simulink subsystem "In_Plane_ModelArchitecture"  (R2025b)
settings: Solver=VariableStepAuto  StartTime=0.0  StopTime=10.0  RelTol=1e-3
undefined symbols (not defined in the file or in its folder): AeroLiftCff, AeroLongDrgCff, AeroMotoEffctArea, AeroPitchMomentCff, AeroPitchMomentLngth, AeroRltWindAngVect, AeroSideFrcCff, AeroYawMomentCff, aMode, BrkFrntBrkActrBore, BrkFrntBrkActrPrsBpt, BrkFrntBrkPadMeanRadius, BrkFrntBrkTrqTbl, BrkFrntIntrnRadius, BrkFrntKinFricCff, BrkFrntPadNum, BrkFrntShoePinToDrumCntrDst, BrkFrntShoePinToFrcAppDst, BrkFrntShoePinToPadEndAng, BrkFrntShoePinToPadStartAng, BrkFrntStcFricCff, BrkFrntWhlSpdBpt, BrkRearBrkActrBore, BrkRearBrkActrPrsBpt, BrkRearBrkPadMeanRadius, BrkRearBrkTrqTbl, BrkRearIntrnRadius, BrkRearKinFricCff, BrkRearPadNum, BrkRearShoePinToDrumCntrDst, BrkRearShoePinToFrcAppDst, BrkRearShoePinToPadEndAng, BrkRearShoePinToPadStartAng, BrkRearStcFricCff, BrkRearWhlSpdBpt, EnvAbsPrs, EnvAirTemp, FrkFrL0, FrmAng0, g, GasCnst, InitFrkLngth, InitMainFrmPitchAng, InitRearArmPitchAng, InitRearCntctPtchLatVel, InitRearCntctPtchLongVel, InitRearCntctPtchY, InitRearCntctPtchZ, InitRollAng, InitYawAng, MotoFrmLngth, MotoFrmMass, MotoGrvty, MotoLatOfst, MotoLongOfst, MotoLowrFrntFrkMass, MotoPtchOfst, MotoRearArmLngth, MotoRearArmMass, MotoRollOfst ... (+25)
libraries: sm_lib x309, nesl_utility_internal x158, nesl_utility x7, autolibsharedcoupling x6, vehdynlibtire x6, sharedtransform x4, shared6dof x1, matrix_library x1, vehdynlibeomcommon x1
(part 2 of 10)

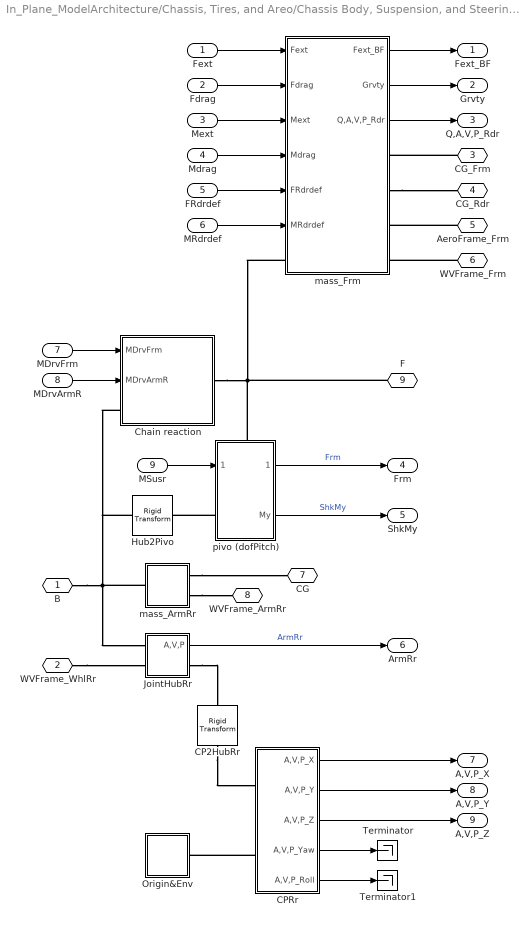
== system In_Plane_ModelArchitecture/Chassis, Tires, and Areo/Chassis Body, Suspension, and Steering/CHASSIS/Chassis body ==
  Fext : Inport
  Fdrag : Inport  Port=2
  Mext : Inport  Port=3
  Mdrag : Inport  Port=4
  FRdrdef : Inport  Port=5
  MRdrdef : Inport  Port=6
  MDrvFrm : Inport  Port=7
  MDrvArmR : Inport  Port=8
  MSusr : Inport  Port=9
  CP2HubRr : sm_lib/Frames and Transforms/Rigid Transform  RotationMethod=None  FollAlignAxisA=+X  BaseAlignAxisA=+Y  FollAlignAxisB=+Y  BaseAlignAxisB=+Z  RotationStandardAxis=+X  RotationAngle=0  RotationAngleUnits=rad  RotationArbitraryAxis=[0 0 1]  RotationSequenceAxes=FollowerAxes  RotationSequence=XYX  RotationSequenceAngles=[0 0 0]  RotationSequenceAnglesUnits=deg  RotationMatrix=[1 0 0; 0 1 0; 0 0 1]  Quaternion=[1 0 0 0]  TranslationMethod=Cartesian  TranslationCartesianOffset=[0 0 -TireRearWhlRadius]  TranslationCartesianOffsetUnits=m  TranslationStandardAxis=+X  TranslationStandardOffset=0  TranslationStandardOffsetUnits=m  TranslationROffset=0  TranslationROffsetUnits=m  TranslationThetaOffset=0  TranslationThetaOffsetUnits=deg  TranslationZOffset=0  TranslationZOffsetUnits=m
  CPRr : Subsystem
  Chain reaction : Subsystem
  Hub2Pivo : sm_lib/Frames and Transforms/Rigid Transform  RotationMethod=None  FollAlignAxisA=+X  BaseAlignAxisA=+Y  FollAlignAxisB=+Y  BaseAlignAxisB=+Z  RotationStandardAxis=+X  RotationAngle=0  RotationAngleUnits=rad  RotationArbitraryAxis=[0 0 1]  RotationSequenceAxes=FollowerAxes  RotationSequence=XYX  RotationSequenceAngles=[0 0 0]  RotationSequenceAnglesUnits=deg  RotationMatrix=[1 0 0; 0 1 0; 0 0 1]  Quaternion=[1 0 0 0]  TranslationMethod=Cartesian  TranslationCartesianOffset=[MotoRearArmLngth, 0, 0]  TranslationCartesianOffsetUnits=m  TranslationStandardAxis=+X  TranslationStandardOffset=0  TranslationStandardOffsetUnits=m  TranslationROffset=0  TranslationROffsetUnits=m  TranslationThetaOffset=0  TranslationThetaOffsetUnits=deg  TranslationZOffset=0  TranslationZOffsetUnits=m
  JointHubRr : Subsystem
  Origin&Env : Subsystem
  Terminator : Terminator
  Terminator1 : Terminator
  mass_ArmRr : Subsystem
  mass_Frm : Subsystem
  pivo (dofPitch) : Subsystem
      settings: PortSchema="{\"entries\":[{\"content\":{\"sides\":[{\"content\":{\"connectorIds\":[\"In1\",\"LConn1\"]},\"type\":\"ConnectorPlacement.EquallySpacedRectSide\",\"uuid\":\"d72cb2b8-1ccd-4071-b85d-9d7143d20021\"},{\"content\":{\"connectorIds\":[\"Out1\",\"Out2\"],\"side\":\"RIGHT\"},\"type\":\"ConnectorPlacement.EquallySpacedRectSide\",\"uuid\":\"efa87c73-460e-407d-bcdf-c587dc7c6fe7\"},{\"content\":{\"connectorIds\":[\"LConn2\"],\"side\":\"TOP\"},\"type\":\"ConnectorPlacement.EquallySpacedRectSide\",\"uuid\":\"615b9486-8369-456a-bccf-ac297a497d74\"}]},\"type\":\"ConnectorPlacement.EquallySpacedConnector\",\"uuid\":\"67d2faff-bcf9-49f8-b2da-dac0f8f5d496\"}],\"packageUris\":[\"http://schema.mathworks.com/mf0/Connector/R2020b\"],\"version\":\"1.0\"}"
  B : PMIOPort  Side=Left
  WVFrame_WhlRr : PMIOPort  Port=2  Side=Left
  CG_Frm : PMIOPort  Port=3  Side=Right
  CG_Rdr : PMIOPort  Port=4  Side=Right
  AeroFrame_Frm : PMIOPort  Port=5  Side=Right
  WVFrame_Frm : PMIOPort  Port=6  Side=Right
  CG : PMIOPort  Port=7  Side=Right
  WVFrame_ArmRr : PMIOPort  Port=8  Side=Right
  F : PMIOPort  Port=9  Side=Right
  Fext_BF : Outport
  Grvty : Outport  Port=2
  Q,A,V,P_Rdr : Outport  Port=3
  Frm : Outport  Port=4
  ShkMy : Outport  Port=5
  ArmRr : Outport  Port=6
  A,V,P_X : Outport  Port=7
  A,V,P_Y : Outport  Port=8
  A,V,P_Z : Outport  Port=9
  wires:
  MRdrdef/1 -> mass_Frm/6(MRdrdef)
  pivo (dofPitch)/1(A,V,P) -> Frm/1  "Frm"
  MDrvFrm/1 -> Chain reaction/1(MDrvFrm)
  mass_Frm/1(Fext_BF) -> Fext_BF/1
  CPRr/2(A,V,P_Y) -> A,V,P_Y/1
  MDrvArmR/1 -> Chain reaction/2(MDrvArmR)
  Mext/1 -> mass_Frm/3(Mext)
  MSusr/1 -> pivo (dofPitch)/1(MSusr)
  CPRr/3(A,V,P_Z) -> A,V,P_Z/1
  pivo (dofPitch)/2(My) -> ShkMy/1  "ShkMy"
  JointHubRr/1(A,V,P) -> ArmRr/1  "ArmRr"
  CPRr/1(A,V,P_X) -> A,V,P_X/1
  Fdrag/1 -> mass_Frm/2(Fdrag)
  Mdrag/1 -> mass_Frm/4(Mdrag)
  FRdrdef/1 -> mass_Frm/5(FRdrdef)
  mass_Frm/3(Q,A,V,P_Rdr) -> Q,A,V,P_Rdr/1
  mass_Frm/2(Grvty) -> Grvty/1
  Fext/1 -> mass_Frm/1(Fext)
  CPRr/4(A,V,P_Yaw) -> Terminator/1
  CPRr/5(A,V,P_Roll) -> Terminator1/1
  connections:
  mass_ArmRr/RConn2 -- WVFrame_ArmRr/RConn1
  mass_ArmRr/RConn1 -- CG/RConn1
  mass_Frm/RConn2 -- CG_Rdr/RConn1
  CG_Frm/RConn1 -- mass_Frm/RConn1
  WVFrame_WhlRr/RConn1 -- JointHubRr/LConn2
  WVFrame_Frm/RConn1 -- mass_Frm/RConn4
  B/RConn1 -- mass_ArmRr/LConn1 -- JointHubRr/LConn1 -- Hub2Pivo/LConn1 -- Chain reaction/LConn1
  JointHubRr/RConn1 -- CP2HubRr/RConn1
  AeroFrame_Frm/RConn1 -- mass_Frm/RConn3
  CP2HubRr/LConn1 -- CPRr/LConn1
  pivo (dofPitch)/LConn1 -- Hub2Pivo/RConn1
  CPRr/LConn2 -- Origin&Env/LConn1
  Chain reaction/RConn1 -- pivo (dofPitch)/LConn2 -- F/RConn1 -- mass_Frm/LConn1

== system In_Plane_ModelArchitecture/Chassis, Tires, and Areo/Chassis Body, Suspension, and Steering/CHASSIS/Sensors ==
  Geom sensor : Subsystem  mask{InitRearCntctPtchZ=InitRearCntctPtchZ, InitMainFrmPitchAng=InitMainFrmPitchAng, InitRearArmPitchAng=InitRearArmPitchAng, InitFrkLngth=InitFrkLngth, MotoUpprFrntFrkOfst=MotoUpprFrntFrkOfst, MotoFrmLngth=MotoFrmLngth, TireRearWhlRadius=TireRearWhlRadius, MotoRearArmLngth=MotoRearArmLngth}
      mask prompts: InitRearCntctPtchZ "Rear contact patch vertical coordinate"; InitMainFrmPitchAng "Pitch angle of main frame"; InitRearArmPitchAng "Pitch angle of rear arm"; InitFrkLngth "Fork length"; MotoUpprFrntFrkOfst "Upper front fork offset"; MotoFrmLngth "Frame length"; TireRearWhlRadius "Rear tire wheel radius"; MotoRearArmLngth "Rear arm length"
      mask init:
      | z_equil        = InitRearCntctPtchZ;
      |     thetafrm_equil = InitMainFrmPitchAng;
      |     thetara_equil  = InitRearArmPitchAng;
      |     df_equil       = InitFrkLngth;
      |     
      |     t2 = cos(thetara_equil);
      |     t3 = cos(thetafrm_equil);
      |     t4 = sin(thetara_equil);
      |     t5 = sin(thetafrm_equil);
      |     t6 = MotoUpprFrntFrkOfst+MotoFrmLngth;
      |     t9 = -TireRearWhlRadius;
      |     t7 = df_equil.*t3;
      |     t8 = df_equil.*t5;
      |     t10 = t3.*t6;
      |     t11 = t5.*t6;
      |     t12 = -t7;
      |     t13 = MotoRearArmLngth+t8+t10;
      |     t16 = t4.*(t7-t11).*(-1.0./2.0);
      |     t17 = (t4.*(t7-t11))./2.0;
      |     t14 = t11+t12;
      |     t15 = (t2.*t13)./2.0;
      |     
      |     ScnOrgnX = t15+t17-MotoRearArmLngth.*t2;
      |     ScnOrgnZ = TireRearWhlRadius-z_equil+MotoRearArmLngth.*t4;
      |     ScnFrntHubX = t15+t17;
      |     ScnFrntHubZ = t9+z_equil-t4.*t13+t2.*(t7-t11);
      |     ScnRearHubX = -t15+t16;
      |     ScnRearHubZ = t9+z_equil;
  HubFr_sensor : Subsystem
  F : PMIOPort  Side=Left
  WVFrame_WhlFr : PMIOPort  Port=2  Side=Right
  HubRr : PMIOPort  Port=3  Side=Left
  HubFr : PMIOPort  Port=4  Side=Left
  pivo : PMIOPort  Port=5  Side=Left
  WhlFrCpX : Outport
  WhlFrCpY : Outport  Port=2
  WhlFrCpZ : Outport  Port=3
  GeomInfo : Outport  Port=4
  wires:
  HubFr_sensor/1(A,V,P_X) -> WhlFrCpX/1  "WhlFrCpX"
  HubFr_sensor/3(A,V,P_Z) -> WhlFrCpZ/1  "WhlFrCpZ"
  HubFr_sensor/2(A,V,P_Y) -> WhlFrCpY/1  "WhlFrCpY"
  Geom sensor/1(GeomInfo) -> GeomInfo/1
  connections:
  Geom sensor/LConn3 -- pivo/RConn1
  Geom sensor/LConn2 -- HubFr/RConn1
  HubRr/RConn1 -- Geom sensor/LConn1
  HubFr_sensor/LConn1 -- F/RConn1
  HubFr_sensor/RConn1 -- WVFrame_WhlFr/RConn1

== system In_Plane_ModelArchitecture/Chassis, Tires, and Areo/Chassis Body, Suspension, and Steering/CHASSIS/Steering and fork ==
  t : Inport
  tExt : Inport  Port=2
  MStrDmpin : Inport  Port=3
  FSusf : Inport  Port=4
  Fork : Subsystem
      settings: PortSchema="{\"entries\":[{\"content\":{\"sides\":[{\"content\":{\"connectorIds\":[\"LConn1\",\"In1\"]},\"type\":\"ConnectorPlacement.EquallySpacedRectSide\",\"uuid\":\"40695b26-fe08-4c8d-a033-d306510a8872\"},{\"content\":{\"connectorIds\":[\"Out1\",\"Out2\",\"RConn1\",\"RConn2\",\"RConn3\",\"RConn4\"],\"side\":\"RIGHT\"},\"type\":\"ConnectorPlacement.EquallySpacedRectSide\",\"uuid\":\"f6b324ba-c46a-4943-898e-93607baa4d0a\"},{\"content\":{\"side\":\"TOP\"},\"type\":\"ConnectorPlacement.EquallySpacedRectSide\",\"uuid\":\"db0879d3-090d-4876-b624-a592cf45df46\"}]},\"type\":\"ConnectorPlacement.EquallySpacedConnector\",\"uuid\":\"71977b15-4414-4fe4-90aa-745731c5184c\"}],\"packageUris\":[\"http://schema.mathworks.com/mf0/Connector/R2020b\"],\"version\":\"1.0\"}"
  Pivo2HP : sm_lib/Frames and Transforms/Rigid Transform  RotationMethod=None  FollAlignAxisA=+X  BaseAlignAxisA=+Y  FollAlignAxisB=+Y  BaseAlignAxisB=+Z  RotationStandardAxis=+X  RotationAngle=0  RotationAngleUnits=rad  RotationArbitraryAxis=[0 0 1]  RotationSequenceAxes=FollowerAxes  RotationSequence=XYX  RotationSequenceAngles=[0 0 0]  RotationSequenceAnglesUnits=deg  RotationMatrix=[1 0 0; 0 1 0; 0 0 1]  Quaternion=[1 0 0 0]  TranslationMethod=Cartesian  TranslationCartesianOffset=[MotoFrmLngth, 0, 0]  TranslationCartesianOffsetUnits=m  TranslationStandardAxis=+X  TranslationStandardOffset=0  TranslationStandardOffsetUnits=m  TranslationROffset=0  TranslationROffsetUnits=m  TranslationThetaOffset=0  TranslationThetaOffsetUnits=deg  TranslationZOffset=0  TranslationZOffsetUnits=m
  Steering : Subsystem
  Unary Minus : UnaryMinus
  B : PMIOPort  Side=Left
  CG_FrkLw : PMIOPort  Port=2  Side=Right
  WVFrame_FrkLw : PMIOPort  Port=3  Side=Right
  WVFrame_FrkUp : PMIOPort  Port=4  Side=Right
  F : PMIOPort  Port=5  Side=Right
  A,V,P : Outport
  FrkFz : Outport  Port=2
  Lfrk : Outport  Port=3
  wires:
  MStrDmpin/1 -> Steering/3(MStrDmpin)
  Fork/2(Lfrk) -> Lfrk/1
  t/1 -> Unary Minus/1
  FSusf/1 -> Fork/1(FSusf)
  tExt/1 -> Steering/2(tExt)
  Fork/1(FrkFz) -> FrkFz/1
  Steering/1(A,V,P) -> A,V,P/1
  Unary Minus/1 -> Steering/1(t)
  connections:
  Pivo2HP/RConn1 -- Steering/LConn1
  B/RConn1 -- Pivo2HP/LConn1
  Fork/RConn1 -- CG_FrkLw/RConn1
  Fork/RConn2 -- WVFrame_FrkLw/RConn1
  Fork/RConn4 -- F/RConn1
  Steering/RConn1 -- Fork/LConn1
  Fork/RConn3 -- WVFrame_FrkUp/RConn1

== system In_Plane_ModelArchitecture/Chassis, Tires, and Areo/Chassis Body, Suspension, and Steering/CHASSIS/Suspension F&M ==
  Lfrk : Inport
  FSusfin : Inport  Port=2
  Frm : Inport  Port=3
  MSusrin : Inport  Port=4
  FrSus F&M : Subsystem  Variant=on  VariantChoicesSpecifier={'Simple_Spring_and_Damper_Suspension'}  VariantControlMode=label  LabelModeActiveChoice=Simple_Spring_and_Damper_Suspension
  RrSus F&M : Subsystem  Variant=on  VariantChoicesSpecifier={'Simple_Spring_and_Damper_Suspension2'}  VariantControlMode=label  LabelModeActiveChoice=Simple_Spring_and_Damper_Suspension2
  FSusf : Outport
  MSusr : Outport  Port=2
  wires:
  RrSus F&M/1(MSusf) -> MSusr/1
  MSusrin/1 -> RrSus F&M/2(MSusrin)
  Lfrk/1 -> FrSus F&M/1(Lfrk)
  FSusfin/1 -> FrSus F&M/2(FSusfin)
  Frm/1 -> RrSus F&M/1(Frm)
  FrSus F&M/1(FSusf) -> FSusf/1

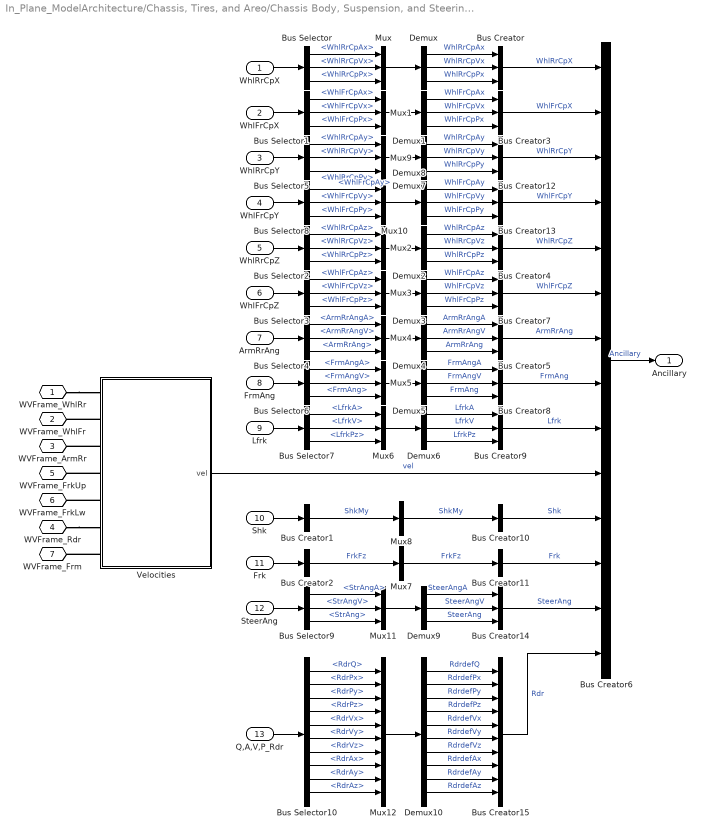
== system In_Plane_ModelArchitecture/Chassis, Tires, and Areo/Chassis Body, Suspension, and Steering/Signal routine/Ancillary_sub ==
  WhlRrCpX : Inport
  WhlFrCpX : Inport  Port=2
  WhlRrCpY : Inport  Port=3
  WhlFrCpY : Inport  Port=4
  WhlRrCpZ : Inport  Port=5
  WhlFrCpZ : Inport  Port=6
  ArmRrAng : Inport  Port=7
  FrmAng : Inport  Port=8
  Lfrk : Inport  Port=9
  Shk : Inport  Port=10
  Frk : Inport  Port=11
  SteerAng : Inport  Port=12
  Q,A,V,P_Rdr : Inport  Port=13
  Bus Creator{,3..5,7..9,12..14} (10 alike) : BusCreator  Inputs=3
  Bus Creator{1..2,10..11} (4 alike) : BusCreator  Inputs=1
  Bus Creator15 : BusCreator  Inputs=10
  Bus Creator6 : BusCreator  Inputs=14
  Bus Selector : BusSelector  OutputSignals=WhlRrCpAx,WhlRrCpVx,WhlRrCpPx
  Bus Selector1 : BusSelector  OutputSignals=WhlFrCpAx,WhlFrCpVx,WhlFrCpPx
  Bus Selector10 : BusSelector  OutputSignals=RdrQ,RdrPx,RdrPy,RdrPz,RdrVx,RdrVy,RdrVz,RdrAx,RdrAy,RdrAz
  Bus Selector2 : BusSelector  OutputSignals=WhlRrCpAz,WhlRrCpVz,WhlRrCpPz
  Bus Selector3 : BusSelector  OutputSignals=WhlFrCpAz,WhlFrCpVz,WhlFrCpPz
  Bus Selector4 : BusSelector  OutputSignals=ArmRrAngA,ArmRrAngV,ArmRrAng
  Bus Selector5 : BusSelector  OutputSignals=WhlRrCpAy,WhlRrCpVy,WhlRrCpPy
  Bus Selector6 : BusSelector  OutputSignals=FrmAngA,FrmAngV,FrmAng
  Bus Selector7 : BusSelector  OutputSignals=LfrkA,LfrkV,LfrkPz
  Bus Selector8 : BusSelector  OutputSignals=WhlFrCpAy,WhlFrCpVy,WhlFrCpPy
  Bus Selector9 : BusSelector  OutputSignals=StrAngA,StrAngV,StrAng
  Demux{,1..9} (10 alike) : Demux  Outputs=3
  Demux10 : Demux  Outputs=10
  Mux{,1..6,9..11} (10 alike) : Mux  Inputs=3
  Mux12 : Mux  Inputs=10
  Mux7 : Mux  Inputs=1
  Mux8 : Mux  Inputs=1
  Velocities : Subsystem
  WVFrame_WhlRr : PMIOPort  Side=Left
  WVFrame_WhlFr : PMIOPort  Port=2  Side=Left
  WVFrame_ArmRr : PMIOPort  Port=3  Side=Left
  WVFrame_Rdr : PMIOPort  Port=4  Side=Left
  WVFrame_FrkUp : PMIOPort  Port=5  Side=Left
  WVFrame_FrkLw : PMIOPort  Port=6  Side=Left
  WVFrame_Frm : PMIOPort  Port=7  Side=Left
  Ancillary : Outport
  wires:
  Bus Creator15/1 -> Bus Creator6/14  "Rdr"
  Demux10/10 -> Bus Creator15/10  "RdrdefAz"
  Demux10/9 -> Bus Creator15/9  "RdrdefAy"
  Demux10/8 -> Bus Creator15/8  "RdrdefAx"
  Demux10/7 -> Bus Creator15/7  "RdrdefVz"
  Demux10/6 -> Bus Creator15/6  "RdrdefVy"
  Demux10/5 -> Bus Creator15/5  "RdrdefVx"
  Demux10/4 -> Bus Creator15/4  "RdrdefPz"
  Demux10/3 -> Bus Creator15/3  "RdrdefPy"
  Demux10/2 -> Bus Creator15/2  "RdrdefPx"
  Demux10/1 -> Bus Creator15/1  "RdrdefQ"
  Mux12/1 -> Demux10/1
  Bus Selector10/10 -> Mux12/10  "<RdrAz>"
  Bus Selector10/9 -> Mux12/9  "<RdrAy>"
  Bus Selector10/8 -> Mux12/8  "<RdrAx>"
  Bus Selector10/7 -> Mux12/7  "<RdrVz>"
  Bus Selector10/6 -> Mux12/6  "<RdrVy>"
  Bus Selector10/5 -> Mux12/5  "<RdrVx>"
  Bus Selector10/4 -> Mux12/4  "<RdrPz>"
  Bus Selector10/3 -> Mux12/3  "<RdrPy>"
  Bus Selector10/2 -> Mux12/2  "<RdrPx>"
  Bus Selector10/1 -> Mux12/1  "<RdrQ>"
  Q,A,V,P_Rdr/1 -> Bus Selector10/1
  Mux11/1 -> Demux9/1
  SteerAng/1 -> Bus Selector9/1
  Bus Selector9/3 -> Mux11/3  "<StrAng>"
  Demux9/3 -> Bus Creator14/3  "SteerAng"
  Demux9/2 -> Bus Creator14/2  "SteerAngV"
  Bus Creator14/1 -> Bus Creator6/13  "SteerAng"
  Bus Selector9/2 -> Mux11/2  "<StrAngV>"
  Demux9/1 -> Bus Creator14/1  "SteerAngA"
  Bus Selector9/1 -> Mux11/1  "<StrAngA>"
  WhlRrCpY/1 -> Bus Selector5/1
  Bus Selector5/1 -> Mux9/1  "<WhlRrCpAy>"
  Bus Selector5/2 -> Mux9/2  "<WhlRrCpVy>"
  Bus Selector5/3 -> Mux9/3  "<WhlRrCpPy>"
  Mux9/1 -> Demux7/1
  Demux7/1 -> Bus Creator12/1  "WhlRrCpAy"
  Demux7/2 -> Bus Creator12/2  "WhlRrCpVy"
  Demux7/3 -> Bus Creator12/3  "WhlRrCpPy"
  Bus Creator12/1 -> Bus Creator6/3  "WhlRrCpY"
  Demux8/3 -> Bus Creator13/3  "WhlFrCpPy"
  Demux8/2 -> Bus Creator13/2  "WhlFrCpVy"
  Demux8/1 -> Bus Creator13/1  "WhlFrCpAy"
  Mux10/1 -> Demux8/1
  Bus Selector8/3 -> Mux10/3  "<WhlFrCpPy>"
  Bus Selector8/2 -> Mux10/2  "<WhlFrCpVy>"
  Bus Selector8/1 -> Mux10/1  "<WhlFrCpAy>"
  Bus Creator13/1 -> Bus Creator6/4  "WhlFrCpY"
  WhlFrCpY/1 -> Bus Selector8/1
  Demux3/3 -> Bus Creator7/3  "WhlFrCpPz"
  Mux7/1 -> Bus Creator11/1  "FrkFz"
  Mux8/1 -> Bus Creator10/1  "ShkMy"
  Bus Creator11/1 -> Bus Creator6/12  "Frk"
  Bus Creator10/1 -> Bus Creator6/11  "Shk"
  Bus Creator9/1 -> Bus Creator6/9  "Lfrk"
  Lfrk/1 -> Bus Selector7/1
  Demux6/3 -> Bus Creator9/3  "LfrkPz"
  Demux6/2 -> Bus Creator9/2  "LfrkV"
  Demux6/1 -> Bus Creator9/1  "LfrkA"
  Mux6/1 -> Demux6/1
  Bus Selector7/3 -> Mux6/3  "<LfrkPz>"
  Bus Selector7/2 -> Mux6/2  "<LfrkV>"
  Bus Selector7/1 -> Mux6/1  "<LfrkA>"
  Bus Creator8/1 -> Bus Creator6/8  "FrmAng"
  FrmAng/1 -> Bus Selector6/1
  Bus Selector6/1 -> Mux5/1  "<FrmAngA>"
  Bus Selector6/2 -> Mux5/2  "<FrmAngV>"
  Bus Selector6/3 -> Mux5/3  "<FrmAng>"
  Mux5/1 -> Demux5/1
  Demux5/1 -> Bus Creator8/1  "FrmAngA"
  Demux5/2 -> Bus Creator8/2  "FrmAngV"
  Demux5/3 -> Bus Creator8/3  "FrmAng"
  Bus Creator5/1 -> Bus Creator6/7  "ArmRrAng"
  Demux4/3 -> Bus Creator5/3  "ArmRrAng"
  Demux4/2 -> Bus Creator5/2  "ArmRrAngV"
  Demux4/1 -> Bus Creator5/1  "ArmRrAngA"
  Mux4/1 -> Demux4/1
  Bus Selector4/3 -> Mux4/3  "<ArmRrAng>"
  Bus Selector4/2 -> Mux4/2  "<ArmRrAngV>"
  Bus Selector4/1 -> Mux4/1  "<ArmRrAngA>"
  ArmRrAng/1 -> Bus Selector4/1
  Bus Creator7/1 -> Bus Creator6/6  "WhlFrCpZ"
  WhlFrCpZ/1 -> Bus Selector3/1
  Mux3/1 -> Demux3/1
  Bus Selector3/1 -> Mux3/1  "<WhlFrCpAz>"
  Bus Selector3/2 -> Mux3/2  "<WhlFrCpVz>"
  Bus Selector3/3 -> Mux3/3  "<WhlFrCpPz>"
  Demux3/1 -> Bus Creator7/1  "WhlFrCpAz"
  Demux3/2 -> Bus Creator7/2  "WhlFrCpVz"
  WhlRrCpZ/1 -> Bus Selector2/1
  Bus Creator4/1 -> Bus Creator6/5  "WhlRrCpZ"
  Demux2/3 -> Bus Creator4/3  "WhlRrCpPz"
  Demux2/2 -> Bus Creator4/2  "WhlRrCpVz"
  Demux2/1 -> Bus Creator4/1  "WhlRrCpAz"
  Mux2/1 -> Demux2/1
  Bus Selector2/3 -> Mux2/3  "<WhlRrCpPz>"
  Bus Selector2/2 -> Mux2/2  "<WhlRrCpVz>"
  Bus Selector2/1 -> Mux2/1  "<WhlRrCpAz>"
  WhlFrCpX/1 -> Bus Selector1/1
  Bus Creator3/1 -> Bus Creator6/2  "WhlFrCpX"
  Bus Selector1/1 -> Mux1/1  "<WhlFrCpAx>"
  Bus Selector1/2 -> Mux1/2  "<WhlFrCpVx>"
  Bus Selector1/3 -> Mux1/3  "<WhlFrCpPx>"
  Mux1/1 -> Demux1/1
  Demux1/1 -> Bus Creator3/1  "WhlFrCpAx"
  Demux1/2 -> Bus Creator3/2  "WhlFrCpVx"
  Demux1/3 -> Bus Creator3/3  "WhlFrCpPx"
  Bus Creator/1 -> Bus Creator6/1  "WhlRrCpX"
  Demux/3 -> Bus Creator/3  "WhlRrCpPx"
  Demux/2 -> Bus Creator/2  "WhlRrCpVx"
  Demux/1 -> Bus Creator/1  "WhlRrCpAx"
  Mux/1 -> Demux/1
  Bus Selector/3 -> Mux/3  "<WhlRrCpPx>"
  Bus Selector/2 -> Mux/2  "<WhlRrCpVx>"
  Bus Selector/1 -> Mux/1  "<WhlRrCpAx>"
  Frk/1 -> Bus Creator2/1
  Bus Creator6/1 -> Ancillary/1  "Ancillary"
  Bus Creator1/1 -> Mux8/1  "ShkMy"
  WhlRrCpX/1 -> Bus Selector/1
  Bus Creator2/1 -> Mux7/1  "FrkFz"
  Velocities/1(vel) -> Bus Creator6/10  "vel"
  Shk/1 -> Bus Creator1/1
  connections:
  Velocities/LConn7 -- WVFrame_Frm/RConn1
  WVFrame_Rdr/RConn1 -- Velocities/LConn6
  WVFrame_WhlRr/RConn1 -- Velocities/LConn1
  Velocities/LConn2 -- WVFrame_WhlFr/RConn1
  Velocities/LConn5 -- WVFrame_FrkLw/RConn1
  Velocities/LConn4 -- WVFrame_FrkUp/RConn1
  Velocities/LConn3 -- WVFrame_ArmRr/RConn1

== system In_Plane_ModelArchitecture/Chassis, Tires, and Areo/Chassis Body, Suspension, and Steering/Signal routine/Geom ==
  GeomInfo : Inport
  SteerAng : Inport  Port=2
  Bus Creator2 : BusCreator  Inputs=5
  Bus Selector : BusSelector  OutputSignals=UE4HubRr_x,UE4HubRr_y,UE4HubRr_z,UE4HubFr_x,UE4HubFr_y,UE4HubFr_z,UE4orig_psi,UE4orig_theta,UE4orig_phi,UE4orig_x,UE4orig_y,UE4orig_z
  Bus Selector1 : BusSelector  OutputSignals=StrAng
  FrmRotInfo : Subsystem
  StrRotInfo : Subsystem
  posFw_l : Subsystem
  posOrigin_w : Subsystem
  posRw_l : Subsystem
  Geom : Outport
  wires:
  StrRotInfo/1(AngStr) -> Bus Creator2/5  "StrRotInfo"
  posOrigin_w/1(xyz) -> Bus Creator2/4  "posOrigin_w"
  FrmRotInfo/1(phi theta psi) -> Bus Creator2/3  "FrmRotInfo"
  posFw_l/1(xyz) -> Bus Creator2/2  "posFw_l"
  posRw_l/1(xyz) -> Bus Creator2/1  "posRw_l"
  Bus Creator2/1 -> Geom/1  "Geom"
  Bus Selector1/1 -> StrRotInfo/1(delta)  "<StrAng>"
  SteerAng/1 -> Bus Selector1/1
  GeomInfo/1 -> Bus Selector/1
  Bus Selector/12 -> posOrigin_w/3(z)  "<UE4orig_z>"
  Bus Selector/1 -> posRw_l/1(x)  "<UE4HubRr_x>"
  Bus Selector/6 -> posFw_l/3(z)  "<UE4HubFr_z>"
  Bus Selector/8 -> FrmRotInfo/2(theta)  "<UE4orig_theta>"
  Bus Selector/2 -> posRw_l/2(y)  "<UE4HubRr_y>"
  Bus Selector/7 -> FrmRotInfo/1(psi)  "<UE4orig_psi>"
  Bus Selector/5 -> posFw_l/2(y)  "<UE4HubFr_y>"
  Bus Selector/9 -> FrmRotInfo/3(phi)  "<UE4orig_phi>"
  Bus Selector/3 -> posRw_l/3(z)  "<UE4HubRr_z>"
  Bus Selector/10 -> posOrigin_w/1(x)  "<UE4orig_x>"
  Bus Selector/4 -> posFw_l/1(x)  "<UE4HubFr_x>"
  Bus Selector/11 -> posOrigin_w/2(y)  "<UE4orig_y>"

== system In_Plane_ModelArchitecture/Chassis, Tires, and Areo/Chassis Body, Suspension, and Steering/Signal routine/Info_sub ==
  Fext_BF : Inport
  Fg : Inport  Port=2
  Fd : Inport  Port=3
  Md : Inport  Port=4
  Mext : Inport  Port=5
  Genrl : Inport  Port=6
  BdyFrm : Subsystem
      settings: PortSchema="{\"entries\":[{\"content\":{\"sides\":[{\"content\":{\"connectorIds\":[\"LConn1\",\"LConn2\",\"In1\",\"In2\",\"In3\",\"In4\",\"In5\"]},\"type\":\"ConnectorPlacement.EquallySpacedRectSide\",\"uuid\":\"e9a88733-aee8-473e-b149-1ae9f507516f\"},{\"content\":{\"connectorIds\":[\"Out1\"],\"side\":\"RIGHT\"},\"type\":\"ConnectorPlacement.EquallySpacedRectSide\",\"uuid\":\"f90722f0-4c29-4561-b113-e7c258b039fb\"},{\"content\":{\"side\":\"TOP\"},\"type\":\"ConnectorPlacement.EquallySpacedRectSide\",\"uuid\":\"6936f8ff-b22e-47c5-8058-1d25fa2e1730\"}]},\"type\":\"ConnectorPlacement.EquallySpacedConnector\",\"uuid\":\"d377e900-b91f-4b9c-8404-46386778306b\"}],\"packageUris\":[\"http://schema.mathworks.com/mf0/Connector/R2020b\"],\"version\":\"1.0\"}"
  Bus Creator1 : BusCreator  Inputs=4
  Ground : Ground
  InertFrm : Subsystem
  F : PMIOPort  Side=Left
  Frame : Outport
  wires:
  Mext/1 -> BdyFrm/5(Mext)
  InertFrm/1(InertFrm) -> Bus Creator1/1  "InertFrm"
  Fg/1 -> BdyFrm/2(Fg)
  BdyFrm/1(BdyFrm) -> Bus Creator1/2  "BdyFrm"
  Bus Creator1/1 -> Frame/1  "Frame"
  Fd/1 -> BdyFrm/3(Fd)
  Md/1 -> BdyFrm/4(Md)
  Ground/1 -> Bus Creator1/3  "PwrInfo"
  Genrl/1 -> Bus Creator1/4  "Genrl"
  Fext_BF/1 -> BdyFrm/1(Fext_BF)
  connections:
  BdyFrm/LConn1 -- F/RConn1 -- InertFrm/LConn2
  BdyFrm/LConn2 -- InertFrm/LConn1

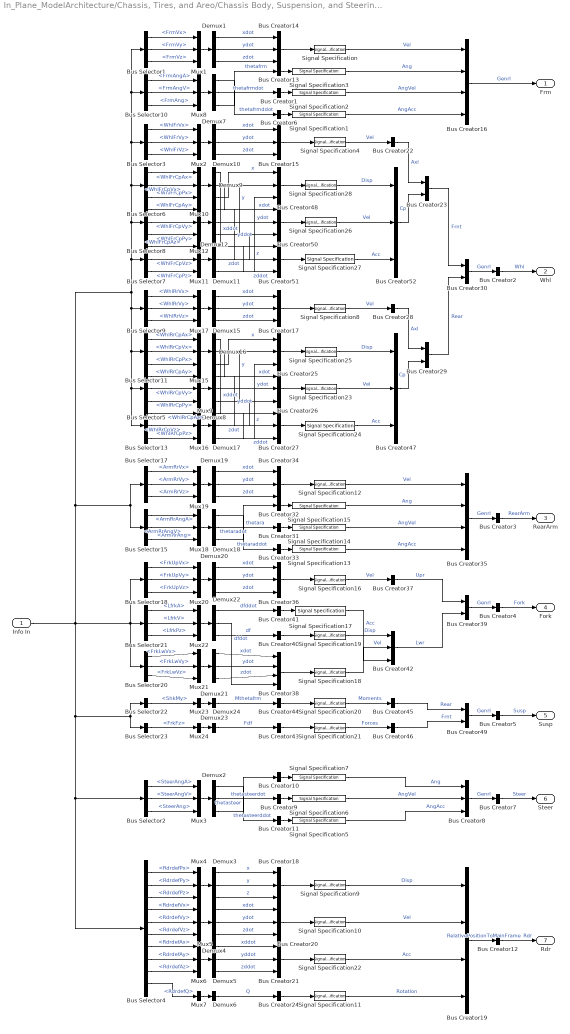
== system In_Plane_ModelArchitecture/Chassis, Tires, and Areo/Chassis Body, Suspension, and Steering/Signal routine/Subsystem Info Busses ==
  Info In : Inport
  Bus Creator{1..7,9..13,22,24,28,31..33,37,40..41,43..46} (25 alike) : BusCreator  Inputs=1
  Bus Creator{8,14..15,17..18,20..21,25..27,34,36,42,47..48,50..52} (18 alike) : BusCreator  Inputs=3
  Bus Creator{16,19,35,38} (4 alike) : BusCreator  Inputs=4
  Bus Creator{23,29..30,39,49} (5 alike) : BusCreator  Inputs=2
  Bus Selector1 : BusSelector  OutputSignals=vel.FrmVx,vel.FrmVy,vel.FrmVz
  Bus Selector10 : BusSelector  OutputSignals=FrmAng.FrmAngA,FrmAng.FrmAngV,FrmAng.FrmAng
  Bus Selector11 : BusSelector  OutputSignals=WhlRrCpX.WhlRrCpAx,WhlRrCpX.WhlRrCpVx,WhlRrCpX.WhlRrCpPx
  Bus Selector13 : BusSelector  OutputSignals=WhlRrCpZ.WhlRrCpAz,WhlRrCpZ.WhlRrCpVz,WhlRrCpZ.WhlRrCpPz
  Bus Selector15 : BusSelector  OutputSignals=ArmRrAng.ArmRrAngA,ArmRrAng.ArmRrAngV,ArmRrAng.ArmRrAng
  Bus Selector17 : BusSelector  OutputSignals=vel.ArmRrVx,vel.ArmRrVy,vel.ArmRrVz
  Bus Selector18 : BusSelector  OutputSignals=vel.FrkUpVx,vel.FrkUpVy,vel.FrkUpVz
  Bus Selector2 : BusSelector  OutputSignals=SteerAng.SteerAngA,SteerAng.SteerAngV,SteerAng.SteerAng
  Bus Selector20 : BusSelector  OutputSignals=vel.FrkLwVx,vel.FrkLwVy,vel.FrkLwVz
  Bus Selector21 : BusSelector  OutputSignals=Lfrk.LfrkA,Lfrk.LfrkV,Lfrk.LfrkPz
  Bus Selector22 : BusSelector  OutputSignals=Shk.ShkMy
  Bus Selector23 : BusSelector  OutputSignals=Frk.FrkFz
  Bus Selector3 : BusSelector  OutputSignals=vel.WhlFrVx,vel.WhlFrVy,vel.WhlFrVz
  Bus Selector4 : BusSelector  OutputSignals=Rdr.RdrdefPx,Rdr.RdrdefPy,Rdr.RdrdefPz,Rdr.RdrdefVx,Rdr.RdrdefVy,Rdr.RdrdefVz,Rdr.RdrdefAx,Rdr.RdrdefAy,Rdr.RdrdefAz,Rdr.RdrdefQ
  Bus Selector5 : BusSelector  OutputSignals=WhlRrCpY.WhlRrCpAy,WhlRrCpY.WhlRrCpVy,WhlRrCpY.WhlRrCpPy
  Bus Selector6 : BusSelector  OutputSignals=WhlFrCpX.WhlFrCpAx,WhlFrCpX.WhlFrCpVx,WhlFrCpX.WhlFrCpPx
  Bus Selector7 : BusSelector  OutputSignals=WhlFrCpZ.WhlFrCpAz,WhlFrCpZ.WhlFrCpVz,WhlFrCpZ.WhlFrCpPz
  Bus Selector8 : BusSelector  OutputSignals=WhlFrCpY.WhlFrCpAy,WhlFrCpY.WhlFrCpVy,WhlFrCpY.WhlFrCpPy
  Bus Selector9 : BusSelector  OutputSignals=vel.WhlRrVx,vel.WhlRrVy,vel.WhlRrVz
  Demux{1..5,7..12,15..22} (19 alike) : Demux  Outputs=3
  Demux23 : Demux  Outputs=1
  Demux24 : Demux  Outputs=1
  Demux6 : Demux  Outputs=1
  Mux{1..6,8..12,15..22} (19 alike) : Mux  Inputs=3
  Mux23 : Mux  Inputs=1
  Mux24 : Mux  Inputs=1
  Mux7 : Mux  Inputs=1
  Signal Specification{,4,8,10,12,16,18,23,26} (9 alike) : SignalSpecification  Unit=m/s
  Signal Specification1 : SignalSpecification  Unit=rad/sec/sec
  Signal Specification{3,7,11,15} (4 alike) : SignalSpecification  Unit=rad
  Signal Specification13 : SignalSpecification  Unit=rad/sec/sec
  Signal Specification14 : SignalSpecification  Unit=rad/sec
  Signal Specification{17,22,24,27} (4 alike) : SignalSpecification  Unit=m/sec/sec
  Signal Specification{9,19,25,28} (4 alike) : SignalSpecification  Unit=m
  Signal Specification2 : SignalSpecification  Unit=rad/sec
  Signal Specification20 : SignalSpecification  Unit=N*m
  Signal Specification21 : SignalSpecification  Unit=N
  Signal Specification5 : SignalSpecification  Unit=rad/sec/sec
  Signal Specification6 : SignalSpecification  Unit=rad/sec
  Frm : Outport
  Whl : Outport  Port=2
  RearArm : Outport  Port=3
  Fork : Outport  Port=4
  Susp : Outport  Port=5
  Steer : Outport  Port=6
  Rdr : Outport  Port=7
  wires:
  Bus Creator52/1 -> Bus Creator23/2  "Cp"
  Demux11/3 -> Bus Creator48/3  "z"
  Bus Selector8/2 -> Mux12/2  "<WhlFrCpVy>"
  Signal Specification27/1 -> Bus Creator52/3  "Acc"
  Demux12/3 -> Bus Creator48/2  "y"
  Bus Selector8/1 -> Mux12/1  "<WhlFrCpAy>"
  Signal Specification26/1 -> Bus Creator52/2  "Vel"
  Bus Selector8/3 -> Mux12/3  "<WhlFrCpPy>"
  Demux11/2 -> Bus Creator50/3  "zdot"
  Demux12/1 -> Bus Creator51/2  "yddot"
  Demux12/2 -> Bus Creator50/2  "ydot"
  Mux12/1 -> Demux12/1
  Bus Selector6/1 -> Mux10/1  "<WhlFrCpAx>"
  Info In/1 -> Bus Selector21/1, Bus Selector18/1, Bus Selector20/1, Bus Selector23/1, Bus Selector22/1, Bus Selector2/1, Bus Selector4/1, Bus Selector9/1, Bus Selector11/1, Bus Selector13/1, Bus Selector5/1, Bus Selector7/1, Bus Selector8/1, Bus Selector6/1, Bus Selector3/1, Bus Selector10/1, Bus Selector1/1, Bus Selector17/1, Bus Selector15/1
  Bus Selector6/3 -> Mux10/3  "<WhlFrCpPx>"
  Demux9/2 -> Bus Creator50/1  "xdot"
  Demux9/1 -> Bus Creator51/1  "xddot"
  Bus Selector7/2 -> Mux11/2  "<WhlFrCpVz>"
  Bus Creator50/1 -> Signal Specification26/1
  Bus Creator48/1 -> Signal Specification28/1
  Bus Creator51/1 -> Signal Specification27/1
  Bus Selector7/1 -> Mux11/1  "<WhlFrCpAz>"
  Demux11/1 -> Bus Creator51/3  "zddot"
  Bus Selector7/3 -> Mux11/3  "<WhlFrCpPz>"
  Signal Specification28/1 -> Bus Creator52/1  "Disp"
  Demux9/3 -> Bus Creator48/1  "x"
  Bus Selector6/2 -> Mux10/2  "<WhlFrCpVx>"
  Mux11/1 -> Demux11/1
  Mux10/1 -> Demux9/1
  Demux8/1 -> Bus Creator27/2  "yddot"
  Demux8/2 -> Bus Creator26/2  "ydot"
  Demux8/3 -> Bus Creator25/2  "y"
  Mux9/1 -> Demux8/1
  Bus Selector5/2 -> Mux9/2  "<WhlRrCpVy>"
  Bus Selector5/1 -> Mux9/1  "<WhlRrCpAy>"
  Bus Selector5/3 -> Mux9/3  "<WhlRrCpPy>"
  Mux15/1 -> Demux16/1
  Signal Specification24/1 -> Bus Creator47/3  "Acc"
  Demux16/2 -> Bus Creator26/1  "xdot"
  Bus Creator47/1 -> Bus Creator29/2  "Cp"
  Mux16/1 -> Demux17/1
  Demux16/3 -> Bus Creator25/1  "x"
  Signal Specification25/1 -> Bus Creator47/1  "Disp"
  Bus Selector13/3 -> Mux16/3  "<WhlRrCpPz>"
  Demux17/1 -> Bus Creator27/3  "zddot"
  Demux17/3 -> Bus Creator25/3  "z"
  Bus Creator27/1 -> Signal Specification24/1
  Bus Selector11/2 -> Mux15/2  "<WhlRrCpVx>"
  Demux16/1 -> Bus Creator27/1  "xddot"
  Signal Specification23/1 -> Bus Creator47/2  "Vel"
  Demux17/2 -> Bus Creator26/3  "zdot"
  Bus Creator25/1 -> Signal Specification25/1
  Bus Selector13/1 -> Mux16/1  "<WhlRrCpAz>"
  Bus Selector13/2 -> Mux16/2  "<WhlRrCpVz>"
  Bus Creator26/1 -> Signal Specification23/1
  Bus Selector11/1 -> Mux15/1  "<WhlRrCpAx>"
  Bus Selector11/3 -> Mux15/3  "<WhlRrCpPx>"
  Bus Creator24/1 -> Signal Specification11/1
  Bus Selector4/10 -> Mux7/1  "<RdrdefQ>"
  Mux7/1 -> Demux6/1
  Demux6/1 -> Bus Creator24/1  "Q"
  Bus Selector4/9 -> Mux6/3  "<RdrdefAz>"
  Bus Selector4/8 -> Mux6/2  "<RdrdefAy>"
  Bus Selector4/7 -> Mux6/1  "<RdrdefAx>"
  Bus Creator21/1 -> Signal Specification22/1
  Demux5/3 -> Bus Creator21/3  "zddot"
  Demux5/2 -> Bus Creator21/2  "yddot"
  Demux5/1 -> Bus Creator21/1  "xddot"
  Mux6/1 -> Demux5/1
  Bus Selector4/4 -> Mux5/1  "<RdrdefVx>"
  Bus Selector4/6 -> Mux5/3  "<RdrdefVz>"
  Bus Selector4/5 -> Mux5/2  "<RdrdefVy>"
  Mux5/1 -> Demux4/1
  Demux4/1 -> Bus Creator20/1  "xdot"
  Demux4/2 -> Bus Creator20/2  "ydot"
  Demux4/3 -> Bus Creator20/3  "zdot"
  Bus Creator20/1 -> Signal Specification10/1
  Bus Creator18/1 -> Signal Specification9/1
  Demux3/3 -> Bus Creator18/3  "z"
  Demux3/2 -> Bus Creator18/2  "y"
  Demux3/1 -> Bus Creator18/1  "x"
  Mux4/1 -> Demux3/1
  Bus Selector4/3 -> Mux4/3  "<RdrdefPz>"
  Bus Selector4/2 -> Mux4/2  "<RdrdefPy>"
  Bus Selector4/1 -> Mux4/1  "<RdrdefPx>"
  Signal Specification22/1 -> Bus Creator19/3  "Acc"
  Signal Specification11/1 -> Bus Creator19/4  "Rotation"
  Signal Specification10/1 -> Bus Creator19/2  "Vel"
  Signal Specification9/1 -> Bus Creator19/1  "Disp"
  Bus Creator19/1 -> Bus Creator12/1  "RelativePositionToMainFrame"
  Bus Creator12/1 -> Rdr/1  "Rdr"
  Signal Specification5/1 -> Bus Creator8/3  "AngAcc"
  Bus Creator9/1 -> Signal Specification6/1
  Bus Selector2/2 -> Mux3/2  "<SteerAngV>"
  Signal Specification6/1 -> Bus Creator8/2  "AngVel"
  Signal Specification7/1 -> Bus Creator8/1  "Ang"
  Bus Creator10/1 -> Signal Specification7/1
  Bus Creator11/1 -> Signal Specification5/1
  Demux2/2 -> Bus Creator9/1  "thetasteerdot"
  Mux3/1 -> Demux2/1
  Bus Selector2/1 -> Mux3/1  "<SteerAngA>"
  Demux2/1 -> Bus Creator11/1  "thetasteerddot"
  Demux2/3 -> Bus Creator10/1  "thetasteer"
  Bus Selector2/3 -> Mux3/3  "<SteerAng>"
  Bus Creator8/1 -> Bus Creator7/1  "Genrl"
  Bus Creator7/1 -> Steer/1  "Steer"
  Demux21/2 -> Bus Creator38/2  "ydot"
  Bus Selector20/2 -> Mux21/2  "<FrkLwVy>"
  Demux20/2 -> Bus Creator36/2  "ydot"
  Bus Selector18/2 -> Mux20/2  "<FrkUpVy>"
  Demux19/2 -> Bus Creator34/2  "ydot"
  Bus Selector17/2 -> Mux19/2  "<ArmRrVy>"
  Demux15/2 -> Bus Creator17/2  "ydot"
  Bus Selector9/2 -> Mux17/2  "<WhlRrVy>"
  Demux10/2 -> Bus Creator15/2  "ydot"
  Bus Selector3/2 -> Mux2/2  "<WhlFrVy>"
  Demux1/2 -> Bus Creator14/2  "ydot"
  Bus Selector1/2 -> Mux1/2  "<FrmVy>"
  Bus Creator36/1 -> Signal Specification16/1
  Signal Specification/1 -> Bus Creator16/1  "Vel"
  Demux21/1 -> Bus Creator38/1  "xdot"
  Bus Creator43/1 -> Signal Specification21/1
  Bus Selector17/1 -> Mux19/1  "<ArmRrVx>"
  Bus Creator37/1 -> Bus Creator39/1  "Upr"
  Bus Creator31/1 -> Signal Specification14/1
  Signal Specification21/1 -> Bus Creator46/1  "Forces"
  Demux23/1 -> Bus Creator43/1  "Fdf"
  Signal Specification3/1 -> Bus Creator16/2  "Ang"
  Bus Creator5/1 -> Susp/1  "Susp"
  Bus Creator23/1 -> Bus Creator30/1  "Frnt"
  Mux19/1 -> Demux19/1
  Demux15/3 -> Bus Creator17/3  "zdot"
  Demux22/1 -> Bus Creator41/1  "dfddot"
  Bus Creator30/1 -> Bus Creator2/1  "Genrl"
  Bus Creator42/1 -> Bus Creator39/2  "Lwr"
  Demux20/1 -> Bus Creator36/1  "xdot"
  Demux18/3 -> Bus Creator32/1  "thetara"
  Bus Selector1/1 -> Mux1/1  "<FrmVx>"
  Demux18/1 -> Bus Creator33/1  "thetaraddot"
  Signal Specification12/1 -> Bus Creator35/1  "Vel"
  Bus Creator40/1 -> Signal Specification19/1
  Bus Creator22/1 -> Bus Creator23/1  "Axl"
  Bus Selector15/1 -> Mux18/1  "<ArmRrAngA>"
  Demux21/3 -> Bus Creator38/3  "zdot"
  Bus Selector15/3 -> Mux18/3  "<ArmRrAng>"
  Bus Creator45/1 -> Bus Creator49/1  "Rear"
  Bus Creator33/1 -> Signal Specification13/1
  Mux23/1 -> Demux24/1
  Bus Creator49/1 -> Bus Creator5/1  "Genrl"
  Signal Specification2/1 -> Bus Creator16/3  "AngVel"
  Mux24/1 -> Demux23/1
  Demux19/1 -> Bus Creator34/1  "xdot"
  Bus Creator2/1 -> Whl/1  "Whl"
  Bus Selector23/1 -> Mux24/1  "<FrkFz>"
  Demux22/3 -> Bus Creator40/1  "df"
  Bus Selector21/2 -> Mux22/2  "<LfrkV>"
  Signal Specification15/1 -> Bus Creator35/2  "Ang"
  Bus Creator3/1 -> RearArm/1  "RearArm"
  Signal Specification1/1 -> Bus Creator16/4  "AngAcc"
  Bus Creator35/1 -> Bus Creator3/1  "Genrl"
  Bus Creator14/1 -> Signal Specification/1
  Bus Creator6/1 -> Signal Specification1/1
  Mux17/1 -> Demux15/1
  Bus Creator16/1 -> Frm/1  "Genrl"
  Bus Creator41/1 -> Signal Specification17/1
  Demux15/1 -> Bus Creator17/1  "xdot"
  Signal Specification14/1 -> Bus Creator35/3  "AngVel"
  Mux18/1 -> Demux18/1
  Demux18/2 -> Bus Creator31/1  "thetaradot"
  Demux7/1 -> Bus Creator6/1  "thetafrmddot"
  Demux7/3 -> Bus Creator13/1  "thetafrm"
  Bus Creator29/1 -> Bus Creator30/2  "Rear"
  Demux19/3 -> Bus Creator34/3  "zdot"
  Bus Creator44/1 -> Signal Specification20/1
  Demux22/2 -> Bus Creator38/4  "dfdot"
  Bus Creator1/1 -> Signal Specification2/1
  Bus Selector9/1 -> Mux17/1  "<WhlRrVx>"
  Bus Creator13/1 -> Signal Specification3/1
  Bus Selector10/2 -> Mux8/2  "<FrmAngV>"
  Bus Selector18/3 -> Mux20/3  "<FrkUpVz>"
  Signal Specification13/1 -> Bus Creator35/4  "AngAcc"
  Bus Selector10/1 -> Mux8/1  "<FrmAngA>"
  Demux20/3 -> Bus Creator36/3  "zdot"
  Demux10/3 -> Bus Creator15/3  "zdot"
  Mux1/1 -> Demux1/1
  Mux22/1 -> Demux22/1
  Bus Creator15/1 -> Signal Specification4/1
  Bus Creator46/1 -> Bus Creator49/2  "Frnt"
  Signal Specification19/1 -> Bus Creator42/1  "Disp"
  Signal Specification8/1 -> Bus Creator28/1  "Vel"
  Bus Selector21/3 -> Mux22/3  "<LfrkPz>"
  Bus Selector1/3 -> Mux1/3  "<FrmVz>"
  Signal Specification4/1 -> Bus Creator22/1  "Vel"
  Bus Creator38/1 -> Signal Specification18/1
  Bus Creator32/1 -> Signal Specification15/1
  Bus Creator28/1 -> Bus Creator29/1  "Axl"
  Bus Selector3/3 -> Mux2/3  "<WhlFrVz>"
  Bus Selector22/1 -> Mux23/1  "<ShkMy>"
  Demux1/3 -> Bus Creator14/3  "zdot"
  Bus Creator4/1 -> Fork/1  "Fork"
  Mux8/1 -> Demux7/1
  Demux10/1 -> Bus Creator15/1  "xdot"
  Bus Selector17/3 -> Mux19/3  "<ArmRrVz>"
  Signal Specification16/1 -> Bus Creator37/1  "Vel"
  Demux1/1 -> Bus Creator14/1  "xdot"
  Bus Selector9/3 -> Mux17/3  "<WhlRrVz>"
  Bus Selector3/1 -> Mux2/1  "<WhlFrVx>"
  Signal Specification20/1 -> Bus Creator45/1  "Moments"
  Bus Selector20/3 -> Mux21/3  "<FrkLwVz>"
  Bus Selector10/3 -> Mux8/3  "<FrmAng>"
  Bus Selector20/1 -> Mux21/1  "<FrkLwVx>"
  Demux24/1 -> Bus Creator44/1  "Mthetafrm"
  Bus Creator34/1 -> Signal Specification12/1
  Bus Selector21/1 -> Mux22/1  "<LfrkA>"
  Mux2/1 -> Demux10/1
  Bus Creator17/1 -> Signal Specification8/1
  Mux20/1 -> Demux20/1
  Bus Selector18/1 -> Mux20/1  "<FrkUpVx>"
  Bus Creator39/1 -> Bus Creator4/1  "Genrl"
  Bus Selector15/2 -> Mux18/2  "<ArmRrAngV>"
  Signal Specification17/1 -> Bus Creator42/3  "Acc"
  Demux7/2 -> Bus Creator1/1  "thetafrmdot"
  Mux21/1 -> Demux21/1
  Signal Specification18/1 -> Bus Creator42/2  "Vel"

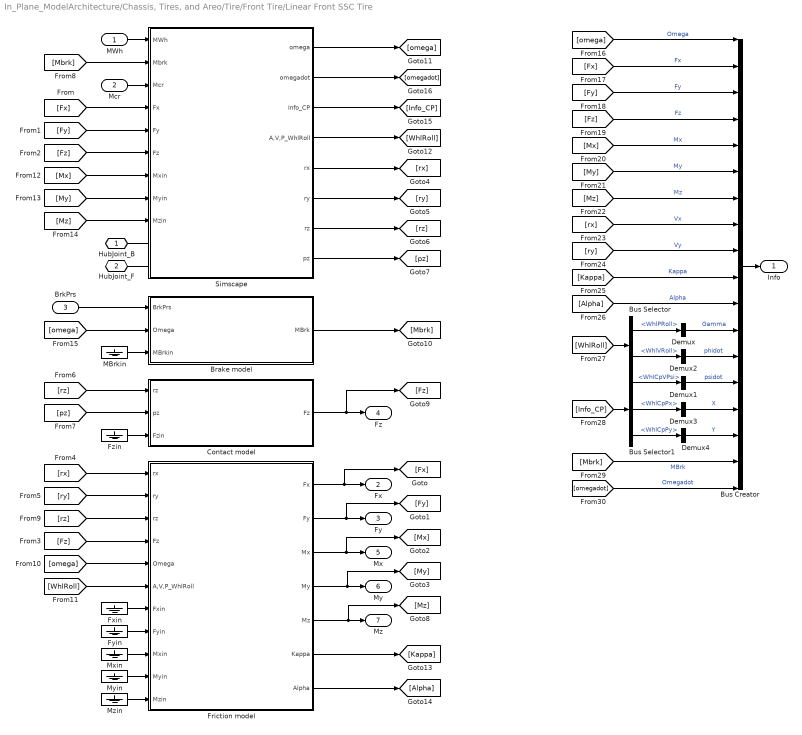
== system In_Plane_ModelArchitecture/Chassis, Tires, and Areo/Tire/Front Tire/Linear Front SSC Tire ==
  MWh : Inport
  Mcr : Inport  Port=2
  BrkPrs : Inport  Port=3
  Brake model : Subsystem  Variant=on  VariantControlMode=label  VariantControl=Choice  LabelModeActiveChoice=MW Brake
  Bus Creator : BusCreator  Inputs=18
  Bus Selector : BusSelector  OutputSignals=WhlPRoll,WhlVRoll
  Bus Selector1 : BusSelector  OutputSignals=WhlCpPsi.WhlCpVPsi,WhlCpX.WhlCpPx,WhlCpY.WhlCpPy
  Contact model : Subsystem  Variant=on  VariantControlMode=label  VariantControl=Choice  LabelModeActiveChoice=Simple spring and damper
  Demux{,1..4} (5 alike) : Demux  Outputs=1
  Friction model : Subsystem  Variant=on  VariantControlMode=label  VariantControl=Choice  LabelModeActiveChoice=Linear
  Fxin : Ground
  Fyin : Ground
  Fzin : Ground
  MBrkin : Ground
  Mxin : Ground
  Myin : Ground
  Mzin : Ground
  Simscape : Subsystem
  HubJoint_B : PMIOPort  Side=Left
  HubJoint_F : PMIOPort  Port=2  Side=Left
  Info : Outport
  Fx : Outport  Port=2
  Fy : Outport  Port=3
  Fz : Outport  Port=4
  Mx : Outport  Port=5
  My : Outport  Port=6
  Mz : Outport  Port=7
  wires:
  [Fx] -> Simscape/4(Fx)
  Friction model/5(Mz) -> [Mz], Mz/1
  Friction model/4(My) -> [My], My/1
  Friction model/3(Mx) -> [Mx], Mx/1
  [Fy] -> Simscape/5(Fy)
  [Fz] -> Simscape/6(Fz)
  Fzin/1 -> Contact model/3(Fzin)
  [rz] -> Contact model/1(rz)
  MWh/1 -> Simscape/1(MWh)
  Mcr/1 -> Simscape/3(Mcr)
  Simscape/3(Info_CP) -> [Info_CP]
  [pz] -> Contact model/2(pz)
  Contact model/1(Fz) -> Fz/1, [Fz]
  Simscape/5(rx) -> [rx]
  Simscape/6(ry) -> [ry]
  Simscape/7(rz) -> [rz]
  Simscape/8(pz) -> [pz]
  [Mbrk] -> Simscape/2(Mbrk)
  Simscape/1(omega) -> [omega]
  Simscape/4(A,V,P_WhlRoll) -> [WhlRoll]
  [rx] -> Friction model/1(rx)
  [ry] -> Friction model/2(ry)
  [rz] -> Friction model/3(rz)
  [Fz] -> Friction model/4(Fz)
  [omega] -> Friction model/5(Omega)
  [WhlRoll] -> Friction model/6(A,V,P_WhlRoll)
  Friction model/1(Fx) -> [Fx], Fx/1
  Friction model/2(Fy) -> Fy/1, [Fy]
  Friction model/6(Kappa) -> [Kappa]
  Friction model/7(Alpha) -> [Alpha]
  Fxin/1 -> Friction model/7(Fxin)
  Fyin/1 -> Friction model/8(Fyin)
  Mxin/1 -> Friction model/9(Mxin)
  Myin/1 -> Friction model/10(Myin)
  Mzin/1 -> Friction model/11(Mzin)
  [Mx] -> Simscape/7(Mxin)
  [My] -> Simscape/8(Myin)
  [Mz] -> Simscape/9(Mzin)
  BrkPrs/1 -> Brake model/1(BrkPrs)
  Brake model/1(MBrk) -> [Mbrk]
  MBrkin/1 -> Brake model/3(MBrkin)
  [omega] -> Brake model/2(Omega)
  [omega] -> Bus Creator/1  "Omega"
  [Fx] -> Bus Creator/2  "Fx"
  [Fy] -> Bus Creator/3  "Fy"
  [Fz] -> Bus Creator/4  "Fz"
  [Mx] -> Bus Creator/5  "Mx"
  [My] -> Bus Creator/6  "My"
  [Mz] -> Bus Creator/7  "Mz"
  [rx] -> Bus Creator/8  "Vx"
  [ry] -> Bus Creator/9  "Vy"
  [Kappa] -> Bus Creator/10  "Kappa"
  [Alpha] -> Bus Creator/11  "Alpha"
  [WhlRoll] -> Bus Selector/1
  Bus Selector/1 -> Demux/1  "<WhlPRoll>"
  [Info_CP] -> Bus Selector1/1
  Bus Selector1/1 -> Demux1/1  "<WhlCpVPsi>"
  Demux/1 -> Bus Creator/12  "Gamma"
  Demux1/1 -> Bus Creator/14  "psidot"
  Bus Creator/1 -> Info/1
  Bus Selector/2 -> Demux2/1  "<WhlVRoll>"
  Demux2/1 -> Bus Creator/13  "phidot"
  Bus Selector1/2 -> Demux3/1  "<WhlCpPx>"
  Bus Selector1/3 -> Demux4/1  "<WhlCpPy>"
  Demux3/1 -> Bus Creator/15  "X"
  Demux4/1 -> Bus Creator/16  "Y"
  [Mbrk] -> Bus Creator/17  "MBrk"
  Simscape/2(omegadot) -> [omegadot]
  [omegadot] -> Bus Creator/18  "Omegadot"
  connections:
  HubJoint_F/RConn1 -- Simscape/LConn2
  HubJoint_B/RConn1 -- Simscape/LConn1

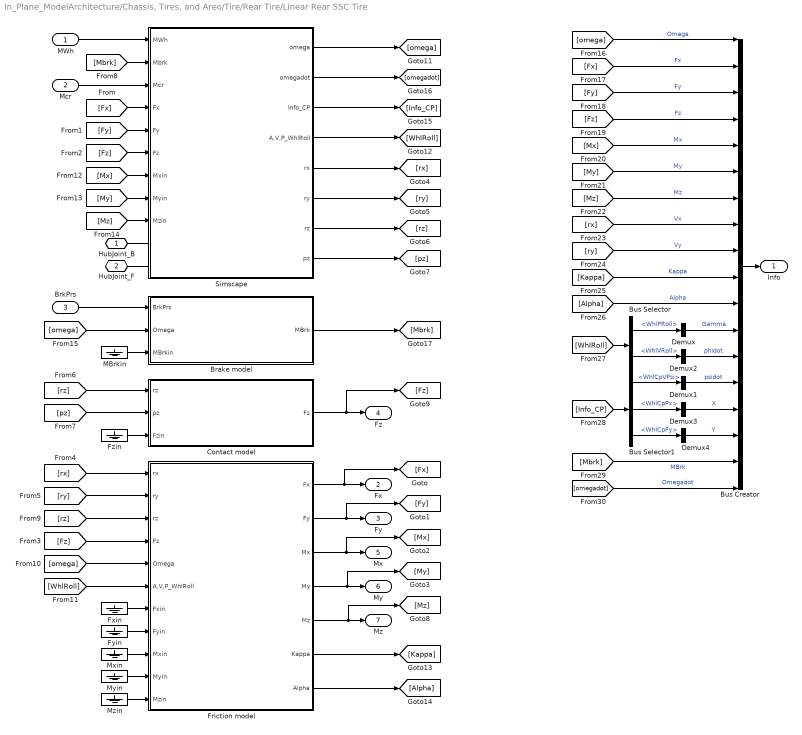
== system In_Plane_ModelArchitecture/Chassis, Tires, and Areo/Tire/Rear Tire/Linear Rear SSC Tire ==
  MWh : Inport
  Mcr : Inport  Port=2
  BrkPrs : Inport  Port=3
  Brake model : Subsystem  Variant=on  VariantControlMode=label  VariantControl=Choice  LabelModeActiveChoice=MW Brake
  Bus Creator : BusCreator  Inputs=18
  Bus Selector : BusSelector  OutputSignals=WhlPRoll,WhlVRoll
  Bus Selector1 : BusSelector  OutputSignals=WhlCpPsi.WhlCpVPsi,WhlCpX.WhlCpPx,WhlCpY.WhlCpPy
  Contact model : Subsystem  Variant=on  VariantControlMode=label  VariantControl=Choice  LabelModeActiveChoice=Simple spring and damper
  Demux{,1..4} (5 alike) : Demux  Outputs=1
  Friction model : Subsystem  Variant=on  VariantControlMode=label  VariantControl=Choice  LabelModeActiveChoice=Linear
  Fxin : Ground
  Fyin : Ground
  Fzin : Ground
  MBrkin : Ground
  Mxin : Ground
  Myin : Ground
  Mzin : Ground
  Simscape : Subsystem
  HubJoint_B : PMIOPort  Side=Left
  HubJoint_F : PMIOPort  Port=2  Side=Left
  Info : Outport
  Fx : Outport  Port=2
  Fy : Outport  Port=3
  Fz : Outport  Port=4
  Mx : Outport  Port=5
  My : Outport  Port=6
  Mz : Outport  Port=7
  wires:
  BrkPrs/1 -> Brake model/1(BrkPrs)
  Brake model/1(MBrk) -> [Mbrk]
  [Fx] -> Simscape/4(Fx)
  Friction model/5(Mz) -> [Mz], Mz/1
  Friction model/4(My) -> [My], My/1
  Friction model/3(Mx) -> [Mx], Mx/1
  [Fy] -> Simscape/5(Fy)
  [Fz] -> Simscape/6(Fz)
  Fzin/1 -> Contact model/3(Fzin)
  [rz] -> Contact model/1(rz)
  MWh/1 -> Simscape/1(MWh)
  Mcr/1 -> Simscape/3(Mcr)
  Simscape/3(Info_CP) -> [Info_CP]
  [pz] -> Contact model/2(pz)
  Contact model/1(Fz) -> Fz/1, [Fz]
  Simscape/5(rx) -> [rx]
  Simscape/6(ry) -> [ry]
  Simscape/7(rz) -> [rz]
  Simscape/8(pz) -> [pz]
  [Mbrk] -> Simscape/2(Mbrk)
  Simscape/1(omega) -> [omega]
  Simscape/4(A,V,P_WhlRoll) -> [WhlRoll]
  [rx] -> Friction model/1(rx)
  [ry] -> Friction model/2(ry)
  [rz] -> Friction model/3(rz)
  [Fz] -> Friction model/4(Fz)
  [omega] -> Friction model/5(Omega)
  [WhlRoll] -> Friction model/6(A,V,P_WhlRoll)
  Friction model/1(Fx) -> [Fx], Fx/1
  Friction model/2(Fy) -> Fy/1, [Fy]
  Friction model/6(Kappa) -> [Kappa]
  Friction model/7(Alpha) -> [Alpha]
  Fxin/1 -> Friction model/7(Fxin)
  Fyin/1 -> Friction model/8(Fyin)
  Mxin/1 -> Friction model/9(Mxin)
  Myin/1 -> Friction model/10(Myin)
  Mzin/1 -> Friction model/11(Mzin)
  [Mx] -> Simscape/7(Mxin)
  [My] -> Simscape/8(Myin)
  [Mz] -> Simscape/9(Mzin)
  MBrkin/1 -> Brake model/3(MBrkin)
  [omega] -> Brake model/2(Omega)
  [omega] -> Bus Creator/1  "Omega"
  [Fx] -> Bus Creator/2  "Fx"
  [Fy] -> Bus Creator/3  "Fy"
  [Fz] -> Bus Creator/4  "Fz"
  [Mx] -> Bus Creator/5  "Mx"
  [My] -> Bus Creator/6  "My"
  [Mz] -> Bus Creator/7  "Mz"
  [rx] -> Bus Creator/8  "Vx"
  [ry] -> Bus Creator/9  "Vy"
  [Kappa] -> Bus Creator/10  "Kappa"
  [Alpha] -> Bus Creator/11  "Alpha"
  [WhlRoll] -> Bus Selector/1
  Bus Selector/1 -> Demux/1  "<WhlPRoll>"
  [Info_CP] -> Bus Selector1/1
  Bus Selector1/1 -> Demux1/1  "<WhlCpVPsi>"
  Demux/1 -> Bus Creator/12  "Gamma"
  Demux1/1 -> Bus Creator/14  "psidot"
  Bus Creator/1 -> Info/1
  Bus Selector/2 -> Demux2/1  "<WhlVRoll>"
  Demux2/1 -> Bus Creator/13  "phidot"
  Bus Selector1/2 -> Demux3/1  "<WhlCpPx>"
  Bus Selector1/3 -> Demux4/1  "<WhlCpPy>"
  Demux3/1 -> Bus Creator/15  "X"
  Demux4/1 -> Bus Creator/16  "Y"
  [Mbrk] -> Bus Creator/17  "MBrk"
  Simscape/2(omegadot) -> [omegadot]
  [omegadot] -> Bus Creator/18  "Omegadot"
  connections:
  HubJoint_F/RConn1 -- Simscape/LConn2
  HubJoint_B/RConn1 -- Simscape/LConn1

== system In_Plane_ModelArchitecture/Chassis, Tires, and Areo/Chassis Body, Suspension, and Steering/CHASSIS/Chassis body/CPRr ==
  " Frame_CPRr" : sm_lib/Body Elements/Graphic  GraphicType=Marker  MarkerShape=Frame  MarkerSize=30  GraphicVisPropType=SimpleVisualProperties  GraphicDiffuseColor=[0.0 0.8 0.2]  GraphicOpacity=1.0  GraphicSpecularColor=[0.5 0.5 0.5 1.0]  GraphicAmbientColor=[0.15 0.15 0.15 1.0]  GraphicEmissiveColor=[0.0 0.0 0.0 1.0]  GraphicShininess=75
  Bus Creator{,1..4} (5 alike) : BusCreator  Inputs=3
  Camera : Subsystem
  Camera_W : Subsystem
  Roll dof : Subsystem  Variant=on  VariantControlMode=label  VariantControl=Choice  LabelModeActiveChoice=Roll locked
  XYZ dof : Subsystem  Variant=on  VariantControlMode=label  VariantControl=Choice  LabelModeActiveChoice=Y locked
  Yaw dof : Subsystem  Variant=on  VariantControlMode=label  VariantControl=Choice  LabelModeActiveChoice=Yaw locked
  F : PMIOPort  Side=Left
  B : PMIOPort  Port=2  Side=Left
  A,V,P_X : Outport
  A,V,P_Y : Outport  Port=2
  A,V,P_Z : Outport  Port=3
  A,V,P_Yaw : Outport  Port=4
  A,V,P_Roll : Outport  Port=5
  wires:
  Roll dof/3(b) -> Bus Creator4/1  "RollA"
  Roll dof/1(q) -> Bus Creator4/3  "RollP"
  Bus Creator4/1 -> A,V,P_Roll/1  "Roll"
  Roll dof/2(w) -> Bus Creator4/2  "RollV"
  Yaw dof/1(q) -> Bus Creator3/3  "YawP"
  Bus Creator3/1 -> A,V,P_Yaw/1  "Yaw"
  Yaw dof/2(w) -> Bus Creator3/2  "YawV"
  Yaw dof/3(b) -> Bus Creator3/1  "YawA"
  XYZ dof/4(py) -> Bus Creator2/3  "WhlRrCpPy"
  Bus Creator2/1 -> A,V,P_Y/1  "WhlRrCpY"
  XYZ dof/5(vy) -> Bus Creator2/2  "WhlRrCpVy"
  XYZ dof/6(ay) -> Bus Creator2/1  "WhlRrCpAy"
  Bus Creator1/1 -> A,V,P_Z/1  "WhlRrCpZ"
  Bus Creator/1 -> A,V,P_X/1  "WhlRrCpX"
  XYZ dof/9(az) -> Bus Creator1/1  "WhlRrCpAz"
  XYZ dof/8(vz) -> Bus Creator1/2  "WhlRrCpVz"
  XYZ dof/3(ax) -> Bus Creator/1  "WhlRrCpAx"
  XYZ dof/7(pz) -> Bus Creator1/3  "WhlRrCpPz"
  XYZ dof/2(vx) -> Bus Creator/2  "WhlRrCpVx"
  XYZ dof/1(px) -> Bus Creator/3  "WhlRrCpPx"
  connections:
  Roll dof/RConn1 -- F/RConn1
  " Frame_CPRr"/RConn1 -- Yaw dof/RConn1 -- Camera/LConn1 -- Roll dof/LConn1
  XYZ dof/RConn1 -- Yaw dof/LConn1 -- Camera_W/LConn1
  B/RConn1 -- XYZ dof/LConn1

== system In_Plane_ModelArchitecture/Chassis, Tires, and Areo/Chassis Body, Suspension, and Steering/CHASSIS/Chassis body/Chain reaction ==
  MDrvFrm : Inport
  MDrvArmR : Inport  Port=2
  External Force and Torque1 : sm_lib/Forces and Torques/External Force and Torque  EnableForceX=off  EnableForceY=off  EnableForceZ=off  EnableForce=off  ForceResolutionFrame=World  EnableTorqueX=off  EnableTorqueY=on  EnableTorqueZ=off  EnableTorque=off  TorqueResolutionFrame=AttachedFrame
  External Force and Torque2 : sm_lib/Forces and Torques/External Force and Torque  EnableForceX=off  EnableForceY=off  EnableForceZ=off  EnableForce=off  ForceResolutionFrame=World  EnableTorqueX=off  EnableTorqueY=on  EnableTorqueZ=off  EnableTorque=off  TorqueResolutionFrame=AttachedFrame
  Graphic : sm_lib/Body Elements/Graphic  GraphicType=Marker  MarkerShape=Frame  MarkerSize=40  GraphicVisPropType=SimpleVisualProperties  GraphicDiffuseColor=[1.0 0.0 0.0]  GraphicOpacity=1.0  GraphicSpecularColor=[0.5 0.5 0.5 1.0]  GraphicAmbientColor=[0.15 0.15 0.15 1.0]  GraphicEmissiveColor=[0.0 0.0 0.0 1.0]  GraphicShininess=75
  Graphic1 : sm_lib/Body Elements/Graphic  GraphicType=Marker  MarkerShape=Frame  MarkerSize=40  GraphicVisPropType=SimpleVisualProperties  GraphicDiffuseColor=[1.0 0.0 0.0]  GraphicOpacity=1.0  GraphicSpecularColor=[0.5 0.5 0.5 1.0]  GraphicAmbientColor=[0.15 0.15 0.15 1.0]  GraphicEmissiveColor=[0.0 0.0 0.0 1.0]  GraphicShininess=75
  Simulink-PS Converter1 : nesl_utility_internal/Simulink-PS Converter  PhysicalDomain=network_engine_domain  SubClassName=ps_input  LeftPortType=input  RightPortType=output  PseudoPeriodic=off  Frequencies=[]  NoiseDistribution=none  NoiseParameters=[]  Unit=N*m  AffineConversion=off  FilteringAndDerivatives=provide  SimscapeFilterOrder=1  InputFilterTimeConstant=0.001  UdotUserProvided=0
  Simulink-PS Converter4 : nesl_utility_internal/Simulink-PS Converter  PhysicalDomain=network_engine_domain  SubClassName=ps_input  LeftPortType=input  RightPortType=output  PseudoPeriodic=off  Frequencies=[]  NoiseDistribution=none  NoiseParameters=[]  Unit=N*m  AffineConversion=off  FilteringAndDerivatives=provide  SimscapeFilterOrder=1  InputFilterTimeConstant=0.001  UdotUserProvided=0
  B : PMIOPort  Side=Left
  F : PMIOPort  Port=2  Side=Right
  wires:
  MDrvArmR/1 -> Simulink-PS Converter4/1
  MDrvFrm/1 -> Simulink-PS Converter1/1
  connections:
  External Force and Torque2/LConn1 -- Simulink-PS Converter4/RConn1
  External Force and Torque1/LConn1 -- Simulink-PS Converter1/RConn1
  External Force and Torque1/RConn1 -- F/RConn1 -- Graphic/RConn1
  Graphic1/RConn1 -- B/RConn1 -- External Force and Torque2/RConn1
